simulink library "pathFollowingControllerExpStateMachineOpenWater_cl"  (R2020a)
settings: Solver=VariableStepAuto  StartTime=0.0  StopTime=10.0  RelTol=1e-3
undefined symbols (not defined in the file or in its folder): a, bScale, courseFollowExp, courseFollowExp_cl, elevatorOL, env, FLIGHTCONTROLLER, fltCtrl, initializeBussesFromBlock, maxBank, perpErrValue, rollMomentKp, rollMomentTau, tanRollKp, tanRollTau, vAppGain, vhcl, vSat, yawMomentKp
libraries: simulink x6, angleBtw2Vecs_ul x4, pathGeometry_ul x3, filteredPIDController_ul x3, eulAng2RotMat_ul x2, tanFrameProjection_ul x2, vectorNormalizer_ul x2, velocityAngle_ul x2, stopwatch_ul x1, dspsigops x1, ctrlAllocMatrixExp_cl x1, vrlib x1
settings Model: Creator=jldanie5  LastModifiedBy=andre
settings DataIOCC: ReturnWorkspaceOutputs=off
settings DebuggingCC: ArithmeticOperatorsInVariantConditions=warning
settings SFSimCC: CustomCodeUndefinedFunction=UseInterfaceOnly

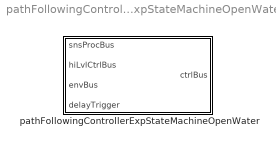
== system pathFollowingControllerExpStateMachineOpenWater_cl ==
  pathFollowingControllerExpStateMachineOpenWater : Subsystem  LoadFcn=initializeBussesFromBlock(gcb)  InitFcn=initializeBussesFromBlock(gcb)  StartFcn=initializeBussesFromBlock(gcb)  VariantControl=strcmpi(FLIGHTCONTROLLER,'pathFollowingControllerMantaBandLin')  mask{initPosForInitSStar=vhcl.initPosVecGnd.Value, fluidDensity=env.water.density.Value, pathCtrl=fltCtrl, aeroStruct=vhcl.struct('OCT.aeroSurf'), thrAttach=vhcl.rBridle_LE.Value, vhcl=vhcl}
      mask prompts: initPosForInitSStar "Initial Position"; fluidDensity "Fluid Density"; pathCtrl "Controller"; aeroStruct "Aerodynamic Structure"; thrAttach "Tether Attach Point"; vhcl "Vehicle"
      settings: MinAlgLoopOccurrences=on
      mask DialogControl Container3 Prompt: courseFollow Params
      mask DialogControl Container4 Prompt: setpointToOutput Params

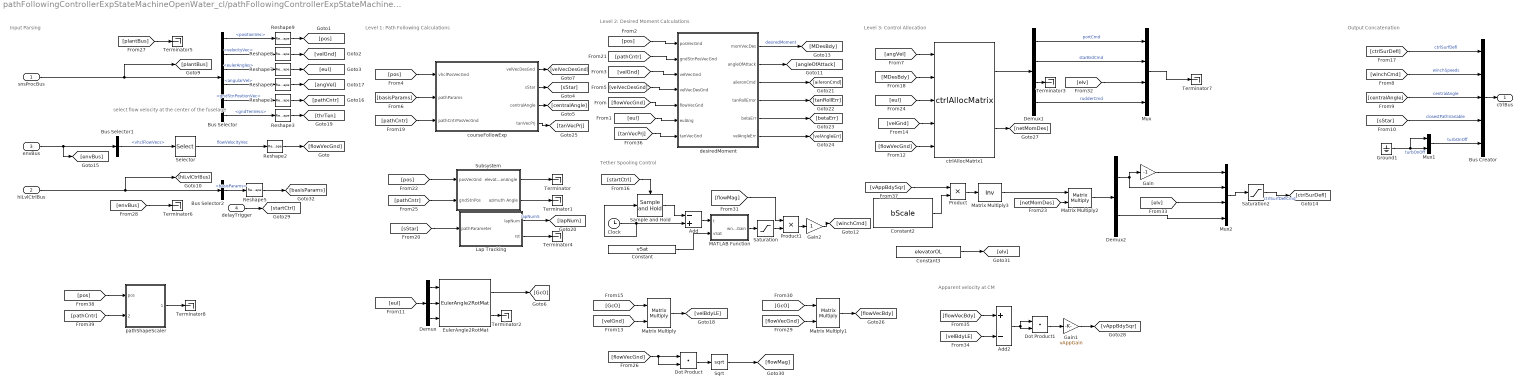
== system pathFollowingControllerExpStateMachineOpenWater_cl/pathFollowingControllerExpStateMachineOpenWater ==
  note: select flow velocity at the center of the fuselage
  note: Level 3: Control Allocation
  note: Output Concatenation
  note: Tether Spooling Control
  note: Level 2: Desired Moment Calculations
  note: Level 1: Path Following Calculations
  note: Input Parsing
  note: Apparent velocity at CM
  snsProcBus : Inport  OutDataTypeStr=Bus: sensorsProcessingBus
  hiLvlCtrlBus : Inport  Port=2  OutDataTypeStr=Bus: hiLvlCtrlBus
  envBus : Inport  Port=3  OutDataTypeStr=Bus: envBus
  delayTrigger : Inport  Port=4
  Add : Sum  Inputs=-+
  Add2 : Sum  Inputs=+-
  Bus Creator : BusCreator  Inputs=5  OutDataTypeStr=Bus: fltCtrlBus
      settings: InheritFromInputs=off
  Bus Selector : BusSelector  OutputSignals=positionVec,velocityVec,eulerAngles,angularVel,gndStnPositionVec,gndTenVecs
  Bus Selector1 : BusSelector  OutputSignals=vhclFlowVecs
  Bus Selector2 : BusSelector  OutputSignals=basisParams
  Clock : Clock
  Constant : Constant  Value=vSat
  Constant2 : Constant  Value=bScale
  Constant3 : Constant  Value=elevatorOL
  Demux : Demux  Outputs=3
  Demux1 : Demux
  Demux2 : Demux  Outputs=2
  Dot Product : DotProduct  InputSameDT=on  OutDataTypeStr=Inherit: Inherit via internal rule
  Dot Product1 : DotProduct  InputSameDT=on  OutDataTypeStr=Inherit: Inherit via internal rule
  EulerAngle2RotMat : eulAng2RotMat_ul/EulerAngle2RotMat  SystemSampleTime=-1  Latency=0  AutoFrameSizeCalculation=off
  Gain : Gain  Gain=-1
  Gain1 : Gain  Gain=vAppGain
  Gain2 : Gain
  Ground1 : Ground
  Lap Tracking : Subsystem
  MATLAB Function : MATLAB Function  TreatAsAtomicUnit=on
  Matrix Multiply : Product  Multiplication=Matrix(*)
  Matrix Multiply1 : Product  Multiplication=Matrix(*)
  Matrix Multiply2 : Product  Multiplication=Matrix(*)
  Matrix Multiply3 : Product  Inputs=/  Multiplication=Matrix(*)
  Mux : Mux
  Mux1 : Mux  Inputs=2
  Mux2 : Mux
  Product : Product
  Product1 : Product
  Reshape{1..3,5..9} (8 alike) : Reshape  OutputDimensionality=Column vector (2-D)
  Sample and Hold : dspsigops/Sample and Hold  trig=Rising edge  initCond=0  latchinput=off
  Saturation : Saturate  UpperLimit=fltCtrl.vSat.Value  LowerLimit=0
  Saturation2 : Saturate  UpperLimit=pathCtrl.controlSigMax.upperLimit.Value  LowerLimit=pathCtrl.controlSigMax.lowerLimit.Value
  Selector : Selector  NumberOfDimensions=2  InputPortWidth=3  IndexOptions=Select all,Index vector (dialog)  Indices=[1 3],5  OutputSizes=1,1
  Sqrt : Sqrt  SaturateOnIntegerOverflow=on
  Subsystem : Subsystem
  Terminator{,1..8} (9 alike) : Terminator
  courseFollowExp : Subsystem  AncestorBlock=courseFollowExp_cl/courseFollowExp
  ctrlAllocMatrix1 : ctrlAllocMatrixExp_cl/ctrlAllocMatrix  aeroStruct=vhcl.struct('OCT.aeroSurf')  fluidDensity=fluidDensity
  desiredMoment : Subsystem
  pathShapeScaler : Subsystem
  ctrlBus : Outport  OutDataTypeStr=Bus: fltCtrlBus  VectorParamsAs1DForOutWhenUnconnected=off
  wires:
  Bus Selector/6 -> Reshape3/1  "<gndTenVecs>"
  Reshape3/1 -> [thrTen]
  courseFollowExp/1(velVecDesGnd) -> [velVecDesGnd]
  snsProcBus/1 -> Bus Selector/1, [plantBus]
  Bus Selector/2 -> Reshape8/1  "<velocityVec>"
  Bus Selector/1 -> Reshape9/1  "<positionVec>"
  Bus Selector/3 -> Reshape7/1  "<eulerAngles>"
  [pos] -> courseFollowExp/1("vhclPosVecGnd ")
  Bus Creator/1 -> ctrlBus/1
  [winchCmd] -> Bus Creator/2  "winchSpeeds"
  courseFollowExp/2(sStar) -> [sStar]
  hiLvlCtrlBus/1 -> [hiLvlCtrlBus], Bus Selector2/1
  [centralAngle] -> Bus Creator/3  "centralAngle"
  [sStar] -> Bus Creator/4  "closestPathVariable"
  courseFollowExp/3(centralAngle) -> [centralAngle]
  desiredMoment/1(momVecDes) -> [MDesBdy]  "desiredMoment"
  Bus Selector/4 -> Reshape6/1  "<angularVel>"
  [angVel] -> ctrlAllocMatrix1/1
  Demux1/3 -> Terminator3/1
  Demux1/1 -> Mux/1  "portCmd"
  Demux1/2 -> Mux/2  "starBrdCmd"
  ctrlAllocMatrix1/1 -> Demux1/1
  [ctrlSurDefl] -> Bus Creator/1  "ctrlSurfDefl"
  Bus Selector2/1 -> Reshape5/1  "<basisParams>"
  Reshape5/1 -> [basisParams]
  Saturation2/1 -> [ctrlSurDefl]  "ctrlSurfDeflCmd"
  Reshape2/1 -> [flowVecGnd]
  Reshape6/1 -> [angVel]
  Reshape7/1 -> [eul]
  Reshape8/1 -> [velGnd]
  Reshape9/1 -> [pos]
  Selector/1 -> Reshape2/1  "flowVelocityVec"
  envBus/1 -> [envBus], Bus Selector1/1
  Bus Selector1/1 -> Selector/1  "<vhclFlowVecs>"
  Reshape1/1 -> [pathCntr]
  Bus Selector/5 -> Reshape1/1  "<gndStnPositionVec>"
  [pathCntr] -> courseFollowExp/3(pathCntrPosVecGnd)
  [pos] -> desiredMoment/1(posVecGnd)
  [pathCntr] -> desiredMoment/2(gndStnPosVecGnd)
  [velGnd] -> desiredMoment/3(velVecGnd)
  [velVecDesGnd] -> desiredMoment/4(velVecDesGnd)
  [eul] -> desiredMoment/6(eulAng)
  [flowVecGnd] -> desiredMoment/5(flowVecGnd)
  [basisParams] -> courseFollowExp/2(pathParams)
  Demux1/4 -> Mux/4  "rudderCmd"
  Mux1/1 -> Bus Creator/5  "turbOnOff"
  [pos] -> Subsystem/1(posVecGnd)
  Subsystem/1(elevationAngle) -> Terminator/1
  Subsystem/2(azimuth Angle) -> Terminator1/1
  [elv] -> Mux/3
  desiredMoment/2(angleOfAttack) -> [angleOfAttack]
  [sStar] -> Lap Tracking/1(pathParameter)
  Lap Tracking/2(rst) -> Terminator4/1
  Lap Tracking/1(lapNum) -> [lapNum]  "lapNumS"
  [plantBus] -> Terminator5/1
  [envBus] -> Terminator6/1
  Constant/1 -> MATLAB Function/2(vSat)
  desiredMoment/3(aileronCmd) -> [aileronCmd]
  Mux/1 -> Terminator7/1
  desiredMoment/4(tanRollError) -> [tanRollErr]
  desiredMoment/5(betaErr) -> [betaErr]
  desiredMoment/6(velAngleErr) -> [velAngleErr]
  courseFollowExp/4(tanVecPrj) -> [tanVecPrj]
  [tanVecPrj] -> desiredMoment/7(tanVecGnd)
  [eul] -> ctrlAllocMatrix1/3
  [flowVecGnd] -> ctrlAllocMatrix1/5
  [MDesBdy] -> ctrlAllocMatrix1/2
  [pathCntr] -> Subsystem/2(gndStnPos)
  Ground1/1 -> Mux1/1, Mux1/2  "turbOnOff"
  [eul] -> Demux/1
  Demux/2 -> EulerAngle2RotMat/2
  Demux/1 -> EulerAngle2RotMat/1
  Demux/3 -> EulerAngle2RotMat/3
  EulerAngle2RotMat/2 -> Terminator2/1
  EulerAngle2RotMat/1 -> [GcO]
  [velGnd] -> Matrix Multiply/2
  [GcO] -> Matrix Multiply/1
  Matrix Multiply/1 -> [velBdyLE]
  Matrix Multiply1/1 -> [flowVecBdy]
  [GcO] -> Matrix Multiply1/1
  [flowVecGnd] -> Matrix Multiply1/2
  Constant2/1 -> Product/2
  Matrix Multiply2/1 -> Demux2/1
  Demux2/1 -> Mux2/2, Gain/1
  Gain/1 -> Mux2/1
  [elv] -> Mux2/3
  Demux2/2 -> Mux2/4
  Add2/1 -> Dot Product1/1, Dot Product1/2
  [flowVecBdy] -> Add2/1
  [velBdyLE] -> Add2/2
  Product/1 -> Matrix Multiply3/1
  Matrix Multiply3/1 -> Matrix Multiply2/1
  ctrlAllocMatrix1/2 -> [netMomDes]
  Dot Product1/1 -> Gain1/1
  [netMomDes] -> Matrix Multiply2/2
  [vAppBdySqr] -> Product/1
  Gain1/1 -> [vAppBdySqr]
  delayTrigger/1 -> [startCtrl]
  [startCtrl] -> Sample and Hold/Trigger
  Clock/1 -> Add/2, Sample and Hold/1
  Sample and Hold/1 -> Add/1
  Add/1 -> MATLAB Function/1(t)
  [flowVecGnd] -> Dot Product/2, Dot Product/1
  Dot Product/1 -> Sqrt/1
  Sqrt/1 -> [flowMag]
  MATLAB Function/1(wnchGain) -> Saturation/1
  [flowMag] -> Product1/1
  Product1/1 -> Gain2/1
  Constant3/1 -> [elv]
  Gain2/1 -> [winchCmd]
  Saturation/1 -> Product1/2
  [pos] -> pathShapeScaler/1(pos)
  [pathCntr] -> pathShapeScaler/2(pathCntr)
  pathShapeScaler/1(basisParams) -> Terminator8/1
  Mux2/1 -> Saturation2/1
  [velGnd] -> ctrlAllocMatrix1/4

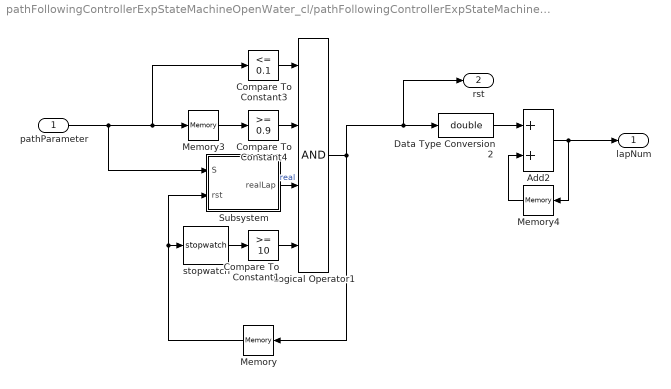
== system pathFollowingControllerExpStateMachineOpenWater_cl/pathFollowingControllerExpStateMachineOpenWater/Lap Tracking ==
  pathParameter : Inport
  Add2 : Sum
  Compare To Constant1 : simulink/Logic and Bit Operations/Compare To Constant  relop=>=  const=10  OutDataTypeStr=boolean
  Compare To Constant3 : simulink/Logic and Bit Operations/Compare To Constant  relop=<=  const=0.1  OutDataTypeStr=boolean
  Compare To Constant4 : simulink/Logic and Bit Operations/Compare To Constant  relop=>=  const=0.9  OutDataTypeStr=boolean
  Data Type Conversion2 : DataTypeConversion  OutDataTypeStr=double
  Logical Operator1 : Logic  Inputs=4  AllPortsSameDT=off  OutDataTypeStr=boolean
  Memory : Memory  InitialCondition=false
  Memory3 : Memory
  Memory4 : Memory
  Subsystem : Subsystem
  stopwatch : stopwatch_ul/stopwatch  SystemSampleTime=-1  Latency=0  AutoFrameSizeCalculation=off
  lapNum : Outport  VectorParamsAs1DForOutWhenUnconnected=off
  rst : Outport  Port=2  VectorParamsAs1DForOutWhenUnconnected=off
  wires:
  Compare To Constant3/1 -> Logical Operator1/1
  Memory3/1 -> Compare To Constant4/1
  Data Type Conversion2/1 -> Add2/1
  Logical Operator1/1 -> rst/1, Data Type Conversion2/1, Memory/1
  Memory4/1 -> Add2/2
  Add2/1 -> lapNum/1, Memory4/1
  Compare To Constant4/1 -> Logical Operator1/2
  pathParameter/1 -> Subsystem/1(S), Compare To Constant3/1, Memory3/1
  stopwatch/1 -> Compare To Constant1/1
  Memory/1 -> Subsystem/2(rst), stopwatch/1
  Compare To Constant1/1 -> Logical Operator1/4
  Subsystem/1(realLap) -> Logical Operator1/3  "real"

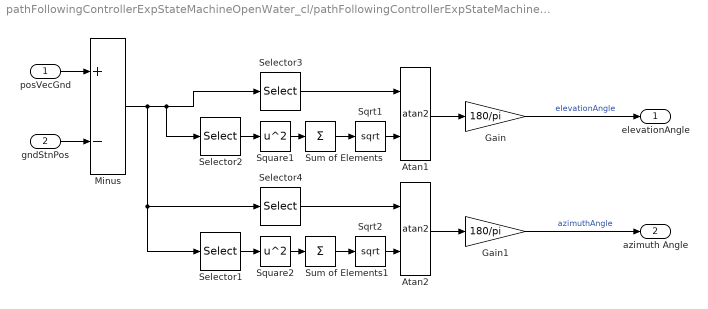
== system pathFollowingControllerExpStateMachineOpenWater_cl/pathFollowingControllerExpStateMachineOpenWater/Subsystem ==
  posVecGnd : Inport
  gndStnPos : Inport  Port=2
  Atan1 : Trigonometry  Operator=atan2
  Atan2 : Trigonometry  Operator=atan2
  Gain : Gain  Gain=180/pi
  Gain1 : Gain  Gain=180/pi
  Minus : Sum  Inputs=+-
  Selector1 : Selector  InputPortWidth=3  IndexOptions=Index vector (dialog)  Indices=1  OutputSizes=1
  Selector2 : Selector  InputPortWidth=3  IndexOptions=Index vector (dialog)  Indices=[1 2]  OutputSizes=1
  Selector3 : Selector  InputPortWidth=3  IndexOptions=Index vector (dialog)  Indices=3  OutputSizes=1
  Selector4 : Selector  InputPortWidth=3  IndexOptions=Index vector (dialog)  Indices=2  OutputSizes=1
  Sqrt1 : Sqrt  SaturateOnIntegerOverflow=on
  Sqrt2 : Sqrt  SaturateOnIntegerOverflow=on
  Square1 : Math  Operator=square  SignedPower=on  SaturateOnIntegerOverflow=on
  Square2 : Math  Operator=square  SignedPower=on  SaturateOnIntegerOverflow=on
  Sum of Elements : Sum  Inputs=+
  Sum of Elements1 : Sum  Inputs=+
  elevationAngle : Outport
  azimuth Angle : Outport  Port=2
  wires:
  Gain1/1 -> azimuth Angle/1  "azimuthAngle"
  Selector4/1 -> Atan2/1
  Sqrt2/1 -> Atan2/2
  Selector1/1 -> Square2/1
  Sum of Elements1/1 -> Sqrt2/1
  Square2/1 -> Sum of Elements1/1
  Atan2/1 -> Gain1/1
  Gain/1 -> elevationAngle/1  "elevationAngle"
  Selector2/1 -> Square1/1
  Atan1/1 -> Gain/1
  Sum of Elements/1 -> Sqrt1/1
  Selector3/1 -> Atan1/1
  Square1/1 -> Sum of Elements/1
  Sqrt1/1 -> Atan1/2
  posVecGnd/1 -> Minus/1
  gndStnPos/1 -> Minus/2
  Minus/1 -> Selector4/1, Selector1/1, Selector2/1, Selector3/1

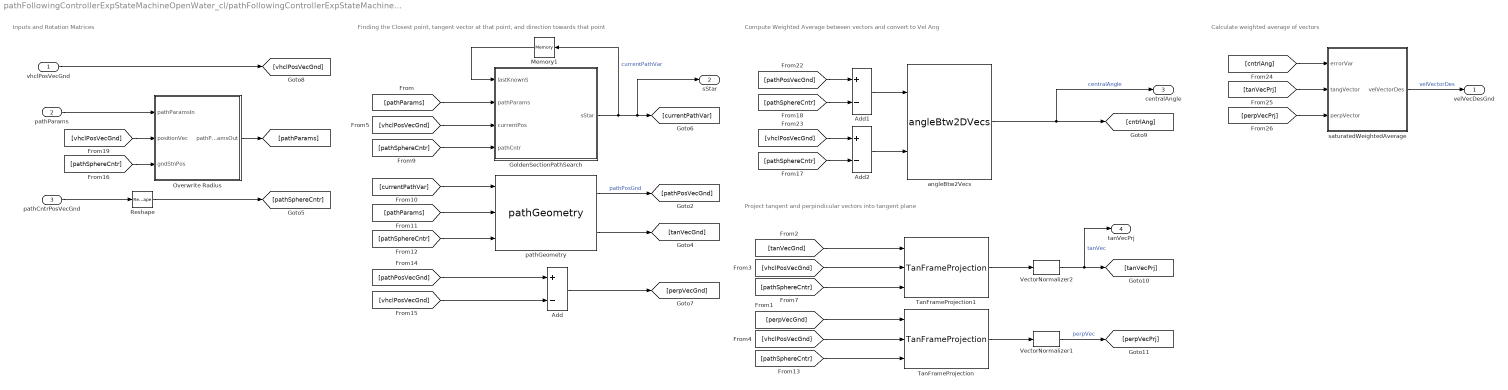
== system pathFollowingControllerExpStateMachineOpenWater_cl/pathFollowingControllerExpStateMachineOpenWater/courseFollowExp ==
  note: Finding the Closest point, tangent vector at that point, and direction towards that point
  note: Inputs and Rotation Matrices
  note: Compute Weighted Average between vectors and convert to Vel Ang
  note: Project tangent and perpindicular vectors into tangent plane
  note: Calculate weighted average of vectors
  "vhclPosVecGnd " : Inport
  pathParams : Inport  Port=2
  pathCntrPosVecGnd : Inport  Port=3
  Add : Sum  Inputs=+-
  Add1 : Sum  Inputs=+-
  Add2 : Sum  Inputs=+-
  GoldenSectionPathSearch : Subsystem  TreatAsAtomicUnit=on
  Memory1 : Memory  InitialCondition=pathCtrl.initPathVar.Value
  Overwrite Radius : Subsystem
  Reshape : Reshape  OutputDimensionality=Column vector (2-D)
  TanFrameProjection : tanFrameProjection_ul/TanFrameProjection  SystemSampleTime=-1  Latency=0  AutoFrameSizeCalculation=off
  TanFrameProjection1 : tanFrameProjection_ul/TanFrameProjection  SystemSampleTime=-1  Latency=0  AutoFrameSizeCalculation=off
  VectorNormalizer1 : vectorNormalizer_ul/VectorNormalizer   SystemSampleTime=-1  Latency=0  AutoFrameSizeCalculation=off
  VectorNormalizer2 : vectorNormalizer_ul/VectorNormalizer   SystemSampleTime=-1  Latency=0  AutoFrameSizeCalculation=off
  angleBtw2Vecs : angleBtw2Vecs_ul/angleBtw2DVecs  SystemSampleTime=-1  Latency=0  AutoFrameSizeCalculation=off
  pathGeometry : pathGeometry_ul/pathGeometry  SystemSampleTime=-1  Latency=0  AutoFrameSizeCalculation=off
  saturatedWeightedAverage : Subsystem  mask{error_upper_lim=perpErrValue}
      mask prompts: error_upper_lim "Value of Error yielding 100% perpendicular"
  velVecDesGnd : Outport  VectorParamsAs1DForOutWhenUnconnected=off
  sStar : Outport  Port=2  VectorParamsAs1DForOutWhenUnconnected=off
  centralAngle : Outport  Port=3  VectorParamsAs1DForOutWhenUnconnected=off
  tanVecPrj : Outport  Port=4
  wires:
  saturatedWeightedAverage/1("velVectorDes ") -> velVecDesGnd/1  "velVectorDes"
  [perpVecPrj] -> saturatedWeightedAverage/3("perpVector ")
  [tanVecPrj] -> saturatedWeightedAverage/2(tangVector)
  [cntrlAng] -> saturatedWeightedAverage/1("errorVar ")
  [pathSphereCntr] -> TanFrameProjection/3
  [pathSphereCntr] -> TanFrameProjection1/3
  [vhclPosVecGnd] -> TanFrameProjection/2
  [vhclPosVecGnd] -> TanFrameProjection1/2
  [tanVecGnd] -> TanFrameProjection1/1
  [perpVecGnd] -> TanFrameProjection/1
  [vhclPosVecGnd] -> Overwrite Radius/2(positionVec)
  [pathSphereCntr] -> Overwrite Radius/3(gndStnPos)
  Add2/1 -> angleBtw2Vecs/2
  Add1/1 -> angleBtw2Vecs/1
  [pathSphereCntr] -> Add1/2
  [pathSphereCntr] -> Add2/2
  [pathSphereCntr] -> GoldenSectionPathSearch/4(pathCntr)
  [pathSphereCntr] -> pathGeometry/3
  Reshape/1 -> [pathSphereCntr]
  pathCntrPosVecGnd/1 -> Reshape/1
  Overwrite Radius/1(pathParamsOut) -> [pathParams]
  pathParams/1 -> Overwrite Radius/1(pathParamsIn)
  TanFrameProjection/1 -> VectorNormalizer1/1
  pathGeometry/2 -> [tanVecGnd]
  [pathPosVecGnd] -> Add/1
  [vhclPosVecGnd] -> Add/2
  Add/1 -> [perpVecGnd]
  Memory1/1 -> GoldenSectionPathSearch/1(lastKnownS)
  GoldenSectionPathSearch/1(sStar) -> [currentPathVar], sStar/1, Memory1/1  "currentPathVar"
  [pathParams] -> GoldenSectionPathSearch/2(pathParams)
  TanFrameProjection1/1 -> VectorNormalizer2/1
  [currentPathVar] -> pathGeometry/1
  [vhclPosVecGnd] -> Add2/1
  angleBtw2Vecs/1 -> centralAngle/1, [cntrlAng]  "centralAngle"
  VectorNormalizer1/1 -> [perpVecPrj]  "perpVec"
  [pathParams] -> pathGeometry/2
  pathGeometry/1 -> [pathPosVecGnd]  "pathPosGnd"
  "vhclPosVecGnd "/1 -> [vhclPosVecGnd]
  [vhclPosVecGnd] -> GoldenSectionPathSearch/3(currentPos)
  VectorNormalizer2/1 -> [tanVecPrj], tanVecPrj/1  "tanVec"
  [pathPosVecGnd] -> Add1/1

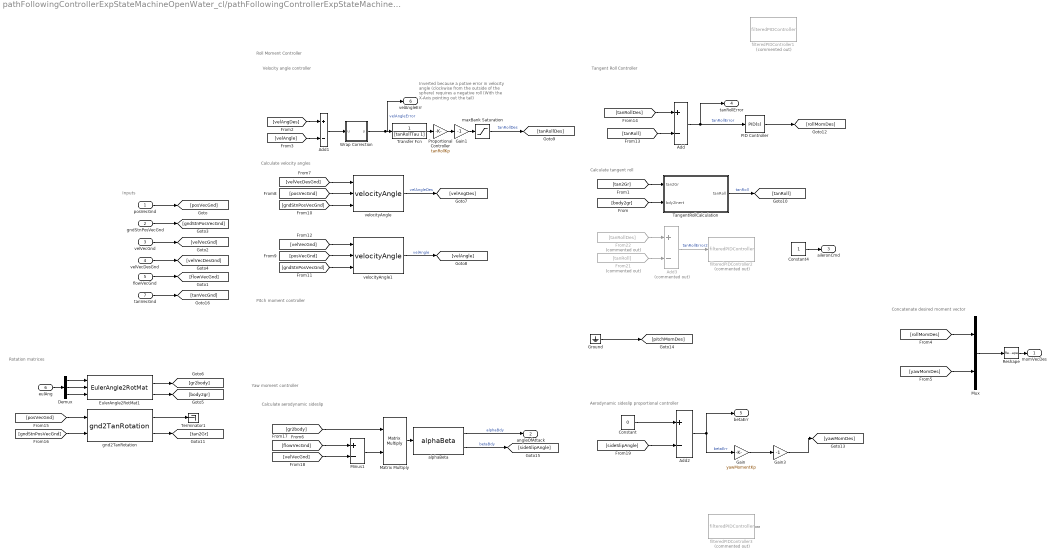
== system pathFollowingControllerExpStateMachineOpenWater_cl/pathFollowingControllerExpStateMachineOpenWater/desiredMoment ==
  note: Yaw moment controller
  note: Pitch moment controller
  note: Inverted because a potive error
      | in velocity angle (clockwise from the
      | outside of the sphere) requires a negative
      | roll (With the X-Axis pointing out the tail)
  note: Velocity angle controller
  note: Inputs
  note: Rotation matrices
  note: Calculate velocity angles
  note: Calculate tangent roll
  note: Tangent Roll Controller
  note: Concatenate desired moment vector
  note: Roll Moment Controller
  note: Aerodynamic sideslip proportional controller
  note: Calculate aerodynamic sideslip
  posVecGnd : Inport
  gndStnPosVecGnd : Inport  Port=2
  velVecGnd : Inport  Port=3
  velVecDesGnd : Inport  Port=4
  flowVecGnd : Inport  Port=5
  eulAng : Inport  Port=6
  tanVecGnd : Inport  Port=7
  Add : Sum  Inputs=+-
  Add1 : Sum  Inputs=+-
  Add2 : Sum  Inputs=+-
  Add3 : Sum  Commented=on  Inputs=+-
  Constant : Constant  Value=0
  Constant4 : Constant
  Demux : Demux  Outputs=3
  EulerAngle2RotMat1 : eulAng2RotMat_ul/EulerAngle2RotMat  SystemSampleTime=-1  Latency=0  AutoFrameSizeCalculation=off
  From21 : From  Commented=on  GotoTag=tanRoll
  From22 : From  Commented=on  GotoTag=tanRollDes
  Gain : Gain  Gain=yawMomentKp
  Gain1 : Gain  Gain=-1
  Gain3 : Gain  Gain=-1
  Ground : Ground
  Matrix Multiply : Product  Multiplication=Matrix(*)
  Minus1 : Sum  Inputs=+-
  Mux : Mux  Inputs=2
  PID Controller : simulink/Continuous/PID Controller  Controller=PID  Form=Parallel  TimeDomain=Continuous-time  UseExternalTs=off  SampleTime=-1  IntegratorMethod=Forward Euler  FilterMethod=Forward Euler  ControllerParametersSource=internal  P=rollMomentKp  I=0  D=fltCtrl.rollMoment.kd.Value  UseFilter=on  N=1/rollMomentTau  TunerSelectOption=Transfer Function Based (PID Tuner App)  InitialConditionSource=internal  InitialConditionForIntegrator=0  InitialConditionForFilter=0  DifferentiatorICPrevScaledInput=0  ExternalReset=none  TrackingMode=off  Kt=1  LimitOutput=off  UpperSaturationLimit=inf  LowerSaturationLimit=-inf  LinearizeAsGain=on  AntiWindupMode=none  Kb=1  POutMin=[]  POutMax=[]  IOutMin=[]  IOutMax=[]  DOutMin=[]  DOutMax=[]  NOutMin=[]  NOutMax=[]  SumOutMin=[]  SumOutMax=[]  SaturationOutMin=[]  SaturationOutMax=[]  PParamMin=[]  PParamMax=[]  IParamMin=[]  IParamMax=[]  DParamMin=[]  DParamMax=[]  NParamMin=[]  NParamMax=[]  KbParamMin=[]  KbParamMax=[]  KtParamMin=[]  KtParamMax=[]  KbOutMin=[]  KbOutMax=[]  KtOutMin=[]  KtOutMax=[]  IntegratorOutMin=[]  IntegratorOutMax=[]  FilterOutMin=[]  FilterOutMax=[]  SumI1OutMin=[]  SumI1OutMax=[]  SumI2OutMin=[]  SumI2OutMax=[]  SumI3OutMin=[]  SumI3OutMax=[]  SumI4OutMin=[]  SumI4OutMax=[]  SumDOutMin=[]  SumDOutMax=[]  DifferentiatorOutMin=[]  DifferentiatorOutMax=[]  FilterDiffOutCoefMin=[]  FilterDiffOutCoefMax=[]  ReciprocalOutMin=[]  ReciprocalOutMax=[]  SumDenOutMin=[]  SumDenOutMax=[]  SumNumOutMin=[]  SumNumOutMax=[]  DivideOutMin=[]  DivideOutMax=[]  UdiffTsProdOutMin=[]  UdiffTsProdOutMax=[]  NTsProdOutMin=[]  NTsProdOutMax=[]  UintegralTsProdOutMin=[]  UintegralTsProdOutMax=[]  UngainTsProdOutMin=[]  UngainTsProdOutMax=[]  IntegratorContinuousStateAttributes=''  IntegratorStateMustResolveToSignalObject=off  IntegratorRTWStateStorageClass=Auto  FilterContinuousStateAttributes=''  FilterStateMustResolveToSignalObject=off  FilterRTWStateStorageClass=Auto  ParallelPVariant=InternalParameters  IdealPVariant=Disabled  IVariant=InternalParameters  DVariant=InternalParameters  IntegratorVariant=Continuous  SatVariant=Disabled  AWVariant=Passthrough  PCopyVariant=Disabled  TRVariant=Disabled  FdbkBlocksVariant=Forward  IdealPFdbkVariant=Disabled  SatFdbkVariant=Disabled  DerivativeFilterVariant=ContFilter  NVariant=InternalParameters  NCopyVariant=Disabled  FilterICVariant=InternalICsFilter  IntegratorICVariant=InternalICs  ExternalResetVariant=Disabled  TRSumVariant=Passthrough  SumFdbkVariant=Disabled  SumVariant=Sum_PID  TsampFilterVariant=InternalTs  TsampNgainVariant=Passthrough  TsampIntegralVariant=Passthrough
  Proportional Controller : Gain  Gain=tanRollKp
  Reshape : Reshape  OutputDimensionality=Column vector (2-D)
  TangentRollCalculation : Subsystem
  Terminator1 : Terminator
  Transfer Fcn : TransferFcn  Denominator=[tanRollTau 1]
  Wrap Correction : Subsystem
  alphaBeta : alphaBeta_ul/alphaBeta  SystemSampleTime=-1  Latency=0  AutoFrameSizeCalculation=off
  filteredPIDController1 : filteredPIDController_ul/filteredPIDController  Commented=on  kp=pathCtrl.rollMoment.kp.Value  ki=0  kd=pathCtrl.rollMoment.kd.Value  Value=pathCtrl.rollMoment.tau.Value  externalReset=none
  filteredPIDController2 : filteredPIDController_ul/filteredPIDController  Commented=on  kp=fltCtrl.rollCtrl.kp.Value  ki=fltCtrl.rollCtrl.ki.Value  kd=fltCtrl.rollCtrl.kd.Value  Value=fltCtrl.rollCtrl.tau.Value  externalReset=none
  filteredPIDController3 : filteredPIDController_ul/filteredPIDController  Commented=on  kp=pathCtrl.yawMoment.kp.Value  ki=0  kd=pathCtrl.yawMoment.kd.Value  Value=pathCtrl.yawMoment.tau.Value  externalReset=none
  gnd2TanRotation : gnd2TanRotation_ul/gnd2TanRotation  SystemSampleTime=-1  Latency=0  AutoFrameSizeCalculation=off
  maxBank Saturation : Saturate  UpperLimit=maxBank  LowerLimit=-maxBank
  velocityAngle : velocityAngle_ul/velocityAngle  SystemSampleTime=-1  Latency=0  AutoFrameSizeCalculation=off
  velocityAngle1 : velocityAngle_ul/velocityAngle  SystemSampleTime=-1  Latency=0  AutoFrameSizeCalculation=off
  momVecDes : Outport  VectorParamsAs1DForOutWhenUnconnected=off
  angleOfAttack : Outport  Port=2  VectorParamsAs1DForOutWhenUnconnected=off
  aileronCmd : Outport  Port=3  VectorParamsAs1DForOutWhenUnconnected=off
  tanRollError : Outport  Port=4
  betaErr : Outport  Port=5
  velAngleErr : Outport  Port=6
  wires:
  [yawMomDes] -> Mux/2
  gnd2TanRotation/1 -> Terminator1/1
  gnd2TanRotation/2 -> [tan2Gr]
  [gndStnPosVecGnd] -> gnd2TanRotation/2
  [posVecGnd] -> gnd2TanRotation/1
  [tanRollDes] -> Add/1
  [tanRoll] -> Add/2
  [velVecGnd] -> velocityAngle1/1
  [gndStnPosVecGnd] -> velocityAngle1/3
  [gndStnPosVecGnd] -> velocityAngle/3
  [posVecGnd] -> velocityAngle1/2
  [posVecGnd] -> velocityAngle/2
  [velVecDesGnd] -> velocityAngle/1
  [velAngle] -> Add1/2
  [velAngDes] -> Add1/1
  velocityAngle1/1 -> [velAngle]  "velAngle"
  velocityAngle/1 -> [velAngDes]  "velAngleDes"
  velVecDesGnd/1 -> [velVecDesGnd]
  gndStnPosVecGnd/1 -> [gndStnPosVecGnd]
  alphaBeta/1 -> angleOfAttack/1  "alphaBdy"
  Add2/1 -> Gain/1, betaErr/1  "betaErr"
  alphaBeta/2 -> [sideSlipAngle]  "betaBdy"
  Matrix Multiply/1 -> alphaBeta/1
  [gr2body] -> Matrix Multiply/1
  [body2gr] -> TangentRollCalculation/2(bdy2Inert)
  EulerAngle2RotMat1/1 -> [gr2body]
  EulerAngle2RotMat1/2 -> [body2gr]
  Demux/2 -> EulerAngle2RotMat1/2
  Demux/1 -> EulerAngle2RotMat1/1
  Demux/3 -> EulerAngle2RotMat1/3
  eulAng/1 -> Demux/1
  [flowVecGnd] -> Minus1/1
  [velVecGnd] -> Minus1/2
  Minus1/1 -> Matrix Multiply/2
  filteredPIDController3/1 -> ?
  TangentRollCalculation/1(tanRoll) -> [tanRoll]  "tanRoll"
  [tan2Gr] -> TangentRollCalculation/1(tan2Gr)
  flowVecGnd/1 -> [flowVecGnd]
  Add1/1 -> Wrap Correction/1(u)
  maxBank Saturation/1 -> [tanRollDes]  "tanRollDes"
  Gain1/1 -> maxBank Saturation/1
  Proportional Controller/1 -> Gain1/1
  Add/1 -> PID Controller/1, tanRollError/1  "tanRollError"
  velVecGnd/1 -> [velVecGnd]
  posVecGnd/1 -> [posVecGnd]
  Ground/1 -> [pitchMomDes]
  Transfer Fcn/1 -> Proportional Controller/1
  Add3/1 -> filteredPIDController2/1  "tanRollError2"
  From21/1 -> Add3/2
  From22/1 -> Add3/1
  tanVecGnd/1 -> [tanVecGnd]
  Wrap Correction/1(y) -> velAngleErr/1, Transfer Fcn/1  "velAngleError"
  Mux/1 -> Reshape/1
  [rollMomDes] -> Mux/1
  Gain3/1 -> [yawMomDes]
  Constant4/1 -> aileronCmd/1
  Reshape/1 -> momVecDes/1
  [sideSlipAngle] -> Add2/2
  PID Controller/1 -> [rollMomDes]
  Gain/1 -> Gain3/1
  Constant/1 -> Add2/1

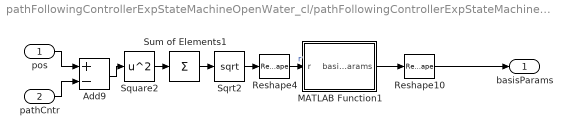
== system pathFollowingControllerExpStateMachineOpenWater_cl/pathFollowingControllerExpStateMachineOpenWater/pathShapeScaler ==
  pos : Inport
  pathCntr : Inport  Port=2
  Add9 : Sum  Inputs=+-
  MATLAB Function1 : MATLAB Function  TreatAsAtomicUnit=on
  Reshape10 : Reshape  OutputDimensionality=Column vector (2-D)
  Reshape4 : Reshape
  Sqrt2 : Sqrt  SaturateOnIntegerOverflow=on
  Square2 : Math  Operator=square  SaturateOnIntegerOverflow=on
  Sum of Elements1 : Sum  Inputs=+
  basisParams : Outport
  wires:
  Sum of Elements1/1 -> Sqrt2/1
  Square2/1 -> Sum of Elements1/1
  MATLAB Function1/1(basisParams) -> Reshape10/1
  pos/1 -> Add9/1
  pathCntr/1 -> Add9/2
  Sqrt2/1 -> Reshape4/1
  Reshape4/1 -> MATLAB Function1/1(r)  "r"
  Reshape10/1 -> basisParams/1
  Add9/1 -> Square2/1

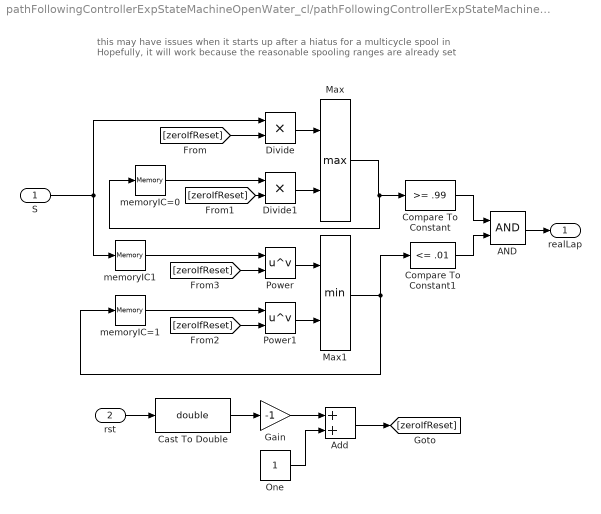
== system pathFollowingControllerExpStateMachineOpenWater_cl/pathFollowingControllerExpStateMachineOpenWater/Lap Tracking/Subsystem ==
  note: this may have issues when it starts up after a hiatus for a multicycle spool in
      | Hopefully, it will work because the reasonable spooling ranges are already set
  S : Inport
  rst : Inport  Port=2
  AND : Logic  AllPortsSameDT=off  OutDataTypeStr=boolean
  Add : Sum
  Cast To Double : DataTypeConversion  OutDataTypeStr=double
  Compare To Constant : simulink/Logic and Bit Operations/Compare To Constant  relop=>=  const=.99  OutDataTypeStr=boolean
  Compare To Constant1 : simulink/Logic and Bit Operations/Compare To Constant  relop=<=  const=.01  OutDataTypeStr=boolean
  Divide : Product  Inputs=**
  Divide1 : Product  Inputs=**
  Gain : Gain  Gain=-1
  Max : MinMax  Function=max  Inputs=2
  Max1 : MinMax  Inputs=2
  One : Constant  OutDataTypeStr=Inherit: Inherit via back propagation
  Power : Math  Operator=pow  SaturateOnIntegerOverflow=on
  Power1 : Math  Operator=pow  SaturateOnIntegerOverflow=on
  memoryIC1 : Memory  InitialCondition=1
  memoryIC=0 : Memory
  memoryIC=1 : Memory  InitialCondition=1
  realLap : Outport
  wires:
  Max1/1 -> Compare To Constant1/1, memoryIC=1/1
  rst/1 -> Cast To Double/1
  S/1 -> Divide/1, memoryIC1/1
  Gain/1 -> Add/1
  Add/1 -> [zeroIfReset]
  One/1 -> Add/2
  Divide/1 -> Max/1
  Max/1 -> memoryIC=0/1, Compare To Constant/1
  Power/1 -> Max1/1
  Power1/1 -> Max1/2
  Cast To Double/1 -> Gain/1
  Compare To Constant/1 -> AND/1
  Compare To Constant1/1 -> AND/2
  AND/1 -> realLap/1
  [zeroIfReset] -> Divide/2
  [zeroIfReset] -> Power/2
  [zeroIfReset] -> Divide1/2
  Divide1/1 -> Max/2
  memoryIC=0/1 -> Divide1/1
  [zeroIfReset] -> Power1/2
  memoryIC=1/1 -> Power1/1
  memoryIC1/1 -> Power/1

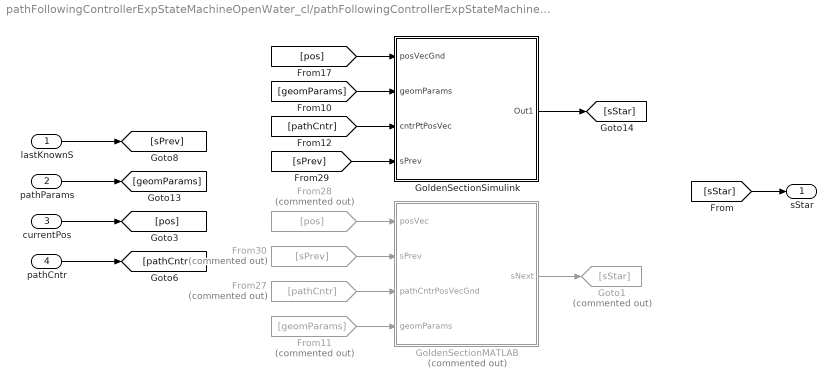
== system pathFollowingControllerExpStateMachineOpenWater_cl/pathFollowingControllerExpStateMachineOpenWater/courseFollowExp/GoldenSectionPathSearch ==
  lastKnownS : Inport
  pathParams : Inport  Port=2
  currentPos : Inport  Port=3
  pathCntr : Inport  Port=4
  From11 : From  Commented=on  GotoTag=geomParams
  From27 : From  Commented=on  GotoTag=pathCntr
  From28 : From  Commented=on  GotoTag=pos
  From30 : From  Commented=on  GotoTag=sPrev
  GoldenSectionMATLAB : MATLAB Function  Commented=on  TreatAsAtomicUnit=on  mask{geomFunc=pathCtrl, searchWidth=0.1, pathVarTol=1e-5}
  GoldenSectionSimulink : Subsystem
  Goto1 : Goto  Commented=on  GotoTag=sStar
  sStar : Outport  InitialOutput=pathCtrl.initPathVar.Value  VectorParamsAs1DForOutWhenUnconnected=off
  wires:
  GoldenSectionSimulink/1(Out1) -> [sStar]
  [sPrev] -> GoldenSectionSimulink/4(sPrev)
  [pathCntr] -> GoldenSectionSimulink/3(cntrPtPosVec)
  [geomParams] -> GoldenSectionSimulink/2(geomParams)
  [pos] -> GoldenSectionSimulink/1(posVecGnd)
  [sStar] -> sStar/1
  lastKnownS/1 -> [sPrev]
  From27/1 -> GoldenSectionMATLAB/3(pathCntrPosVecGnd)
  From30/1 -> GoldenSectionMATLAB/2(sPrev)
  From28/1 -> GoldenSectionMATLAB/1(posVec)
  From11/1 -> GoldenSectionMATLAB/4(geomParams)
  GoldenSectionMATLAB/1(sNext) -> Goto1/1
  pathCntr/1 -> [pathCntr]
  pathParams/1 -> [geomParams]
  currentPos/1 -> [pos]

== system pathFollowingControllerExpStateMachineOpenWater_cl/pathFollowingControllerExpStateMachineOpenWater/courseFollowExp/Overwrite Radius ==
  note: subsystem overwrites the 5th basis parameter with the current radius
      | so that the downstream blocks calculate the path geomatry at the current radius.
  pathParamsIn : Inport
  positionVec : Inport  Port=2
  gndStnPos : Inport  Port=3
  Add : Sum  Inputs=+-
  Assignment : Assignment  NumberOfDimensions=2  DiagnosticForDimensions=Warning  IndexOptions=Index vector (dialog),Assign all  Indices=5,5  OutputSizes=1,1
  Dot Product : DotProduct  InputSameDT=on  OutDataTypeStr=Inherit: Inherit via internal rule
  Sqrt : Sqrt  SaturateOnIntegerOverflow=on
  pathParamsOut : Outport  VectorParamsAs1DForOutWhenUnconnected=off
  wires:
  gndStnPos/1 -> Add/2
  positionVec/1 -> Add/1
  pathParamsIn/1 -> Assignment/1
  Sqrt/1 -> Assignment/2
  Assignment/1 -> pathParamsOut/1
  Dot Product/1 -> Sqrt/1
  Add/1 -> Dot Product/1, Dot Product/2

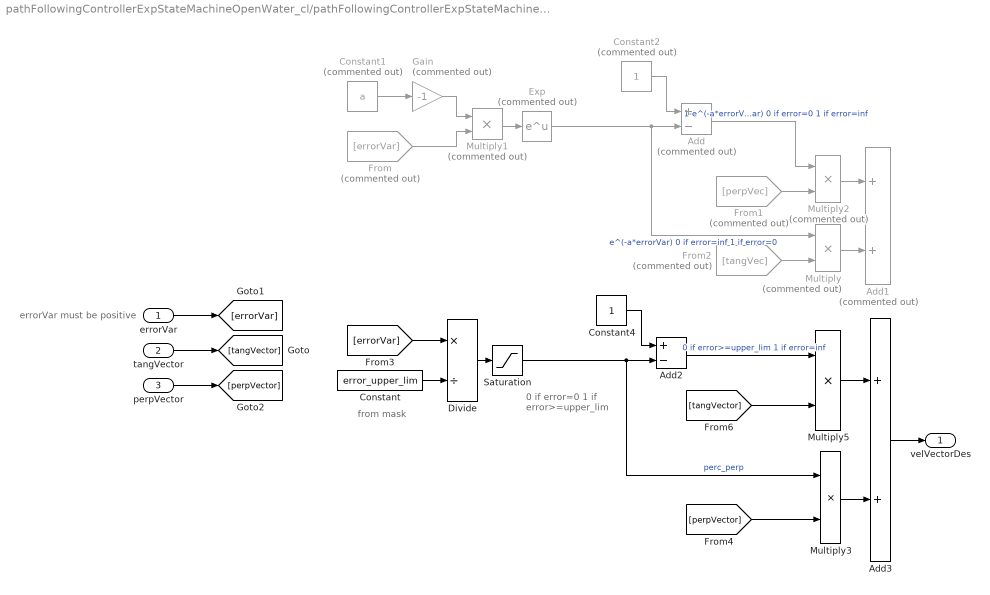
== system pathFollowingControllerExpStateMachineOpenWater_cl/pathFollowingControllerExpStateMachineOpenWater/courseFollowExp/saturatedWeightedAverage ==
  note: 0 if error=0
      | 1 if error>=upper_lim
  note: from mask
  note: errorVar must be positive
  "errorVar " : Inport
  tangVector : Inport  Port=2
  "perpVector " : Inport  Port=3
  Add : Sum  Commented=on  Inputs=+-
  Add1 : Sum  Commented=on
  Add2 : Sum  Inputs=+-
  Add3 : Sum
  Constant : Constant  Value=error_upper_lim
  Constant1 : Constant  Commented=on  Value=a
  Constant2 : Constant  Commented=on
  Constant4 : Constant
  Divide : Product  Inputs=*/
  Exp : Math  Commented=on  SignedPower=on  SaturateOnIntegerOverflow=on
  From : From  Commented=on  GotoTag=errorVar
  From1 : From  Commented=on  GotoTag=perpVec
  From2 : From  Commented=on  GotoTag=tangVec
  Gain : Gain  Commented=on  Gain=-1
  Multiply : Product  Commented=on
  Multiply1 : Product  Commented=on
  Multiply2 : Product  Commented=on
  Multiply3 : Product
  Multiply5 : Product
  Saturation : Saturate  UpperLimit=1  LowerLimit=0
  "velVectorDes " : Outport  VectorParamsAs1DForOutWhenUnconnected=off
  wires:
  tangVector/1 -> [tangVector]
  Constant1/1 -> Gain/1
  Gain/1 -> Multiply1/1
  Multiply1/1 -> Exp/1
  Exp/1 -> Multiply/1, Add/2  "e^(-a*errorVar) 0 if error=inf 1 if error=0"
  Constant2/1 -> Add/1
  Add/1 -> Multiply2/1  "1-e^(-a*errorVar) 0 if error=0 1 if error=inf"
  "errorVar "/1 -> [errorVar]
  "perpVector "/1 -> [perpVector]
  From/1 -> Multiply1/2
  Multiply2/1 -> Add1/1
  Multiply/1 -> Add1/2
  From1/1 -> Multiply2/2
  From2/1 -> Multiply/2
  Constant4/1 -> Add2/1
  Saturation/1 -> Multiply3/1, Add2/2  "perc_perp"
  Add3/1 -> "velVectorDes "/1
  Multiply3/1 -> Add3/2
  Multiply5/1 -> Add3/1
  Add2/1 -> Multiply5/1  "0 if error>=upper_lim 1 if error=inf"
  [errorVar] -> Divide/1
  Constant/1 -> Divide/2
  Divide/1 -> Saturation/1
  [tangVector] -> Multiply5/2
  [perpVector] -> Multiply3/2

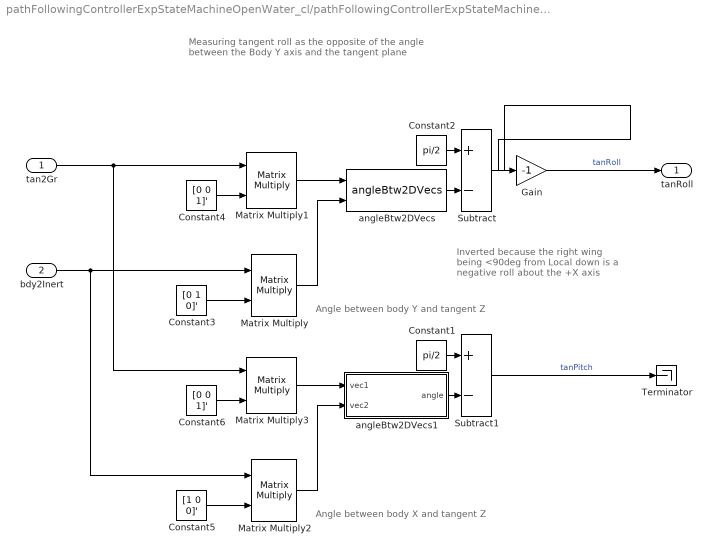
== system pathFollowingControllerExpStateMachineOpenWater_cl/pathFollowingControllerExpStateMachineOpenWater/desiredMoment/TangentRollCalculation ==
  note: Angle between body X and tangent Z
  note: Inverted because the right wing
      | being <90deg from Local down
      | is a negative roll about the +X axis
  note: Angle between body Y and tangent Z
  note: Measuring tangent roll as the opposite
      | of the angle between the Body Y axis
      | and the tangent plane
  tan2Gr : Inport
  bdy2Inert : Inport  Port=2
  Constant1 : Constant  Value=pi/2
  Constant2 : Constant  Value=pi/2
  Constant3 : Constant  Value=[0 1 0]'
  Constant4 : Constant  Value=[0 0 1]'
  Constant5 : Constant  Value=[1 0 0]'
  Constant6 : Constant  Value=[0 0 1]'
  Gain : Gain  Gain=-1
  Matrix Multiply{,1..3} (4 alike) : Product  Multiplication=Matrix(*)
  Subtract : Sum  Inputs=+-
  Subtract1 : Sum  Inputs=+-
  Terminator : Terminator
  angleBtw2DVecs : angleBtw2Vecs_ul/angleBtw2DVecs  SystemSampleTime=-1  Latency=0  AutoFrameSizeCalculation=off
  angleBtw2DVecs1 : Subsystem
  tanRoll : Outport  VectorParamsAs1DForOutWhenUnconnected=off
  wires:
  Constant5/1 -> Matrix Multiply2/2
  angleBtw2DVecs1/1(angle) -> Subtract1/2
  Constant1/1 -> Subtract1/1
  Matrix Multiply3/1 -> angleBtw2DVecs1/1(vec1)
  Constant6/1 -> Matrix Multiply3/2
  Matrix Multiply2/1 -> angleBtw2DVecs1/2(vec2)
  tan2Gr/1 -> Matrix Multiply1/1, Matrix Multiply3/1
  Subtract1/1 -> Terminator/1  "tanPitch"
  bdy2Inert/1 -> Matrix Multiply/1, Matrix Multiply2/1
  Gain/1 -> tanRoll/1  "tanRoll"
  Matrix Multiply/1 -> angleBtw2DVecs/2
  Constant4/1 -> Matrix Multiply1/2
  Matrix Multiply1/1 -> angleBtw2DVecs/1
  Constant2/1 -> Subtract/1
  angleBtw2DVecs/1 -> Subtract/2
  Constant3/1 -> Matrix Multiply/2
  Subtract/1 -> Gain/1

== system pathFollowingControllerExpStateMachineOpenWater_cl/pathFollowingControllerExpStateMachineOpenWater/desiredMoment/Wrap Correction ==
  note: output = mod(input-pi,2*pi)-pi
      | wraps output to -pi to pi
      |
      | ex) 1.5*pi will become -.5pi
      | 	and -1.5pi will become .5pi
      |
      | to visualize, plot the fuction above
  u : Inport
  Add1 : Sum  Inputs=+-
  Add2 : Sum  Inputs=+-
  Constant1 : Constant  Value=pi
  Constant2 : Constant  Value=2*pi
  Constant3 : Constant  Value=pi
  Mod : Math  Operator=mod  SignedPower=on  SaturateOnIntegerOverflow=on
  y : Outport  VectorParamsAs1DForOutWhenUnconnected=off
  wires:
  Add2/1 -> y/1
  Constant3/1 -> Add2/2
  Mod/1 -> Add2/1  "always_pos"
  Constant2/1 -> Mod/2
  Add1/1 -> Mod/1
  Constant1/1 -> Add1/2
  u/1 -> Add1/1

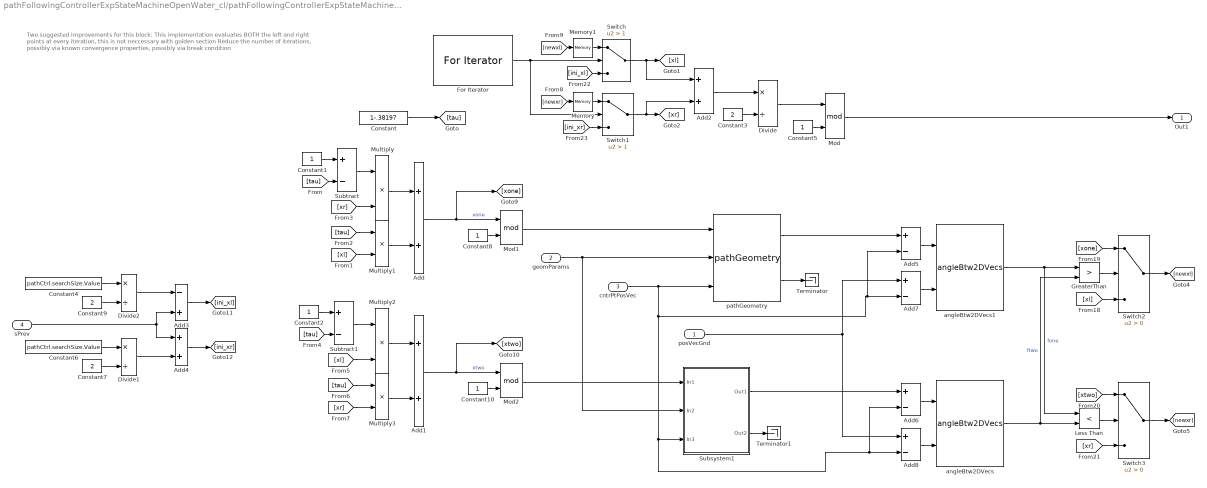
== system pathFollowingControllerExpStateMachineOpenWater_cl/pathFollowingControllerExpStateMachineOpenWater/courseFollowExp/GoldenSectionPathSearch/GoldenSectionSimulink ==
  note: Two suggested improvements for this block:
      | This implementation evaluates BOTH the left and right points at every iteration, this is not neccessary with golden section
      | Reduce the number of iterations, possibly via known convergence properties, possibly via break condition
  posVecGnd : Inport
  geomParams : Inport  Port=2
  cntrPtPosVec : Inport  Port=3
  sPrev : Inport  Port=4
  Add{,1..2,4} (4 alike) : Sum
  Add3 : Sum  Inputs=-+
  Add{5..8} (4 alike) : Sum  Inputs=+-
  Constant : Constant  Value=1-.38197
  Constant{1..2,5,8,10} (5 alike) : Constant
  Constant3 : Constant  Value=2
  Constant4 : Constant  Value=pathCtrl.searchSize.Value
  Constant6 : Constant  Value=pathCtrl.searchSize.Value
  Constant7 : Constant  Value=2
  Constant9 : Constant  Value=2
  Divide : Product  Inputs=*/
  Divide1 : Product  Inputs=*/
  Divide2 : Product  Inputs=*/
  For Iterator : ForIterator  IterationLimit=25
  GreaterThan : RelationalOperator  Operator=>  OutDataTypeStr=boolean  RndMeth=Simplest
  Less Than : RelationalOperator  Operator=<  OutDataTypeStr=boolean  RndMeth=Simplest
  Memory : Memory  InheritSampleTime=on
  Memory1 : Memory  InheritSampleTime=on
  Mod : Math  Operator=mod  SignedPower=on  SaturateOnIntegerOverflow=on
  Mod1 : Math  Operator=mod  SignedPower=on  SaturateOnIntegerOverflow=on
  Mod2 : Math  Operator=mod  SignedPower=on  SaturateOnIntegerOverflow=on
  Multiply{,1..3} (4 alike) : Product
  Subsystem1 : Subsystem
  Subtract : Sum  Inputs=+-
  Subtract1 : Sum  Inputs=+-
  Switch : Switch  Criteria=u2 > Threshold  Threshold=1
  Switch1 : Switch  Criteria=u2 > Threshold  Threshold=1
  Switch2 : Switch  Criteria=u2 > Threshold
  Switch3 : Switch  Criteria=u2 > Threshold
  Terminator : Terminator
  Terminator1 : Terminator
  angleBtw2DVecs : angleBtw2Vecs_ul/angleBtw2DVecs  SystemSampleTime=-1  Latency=0  AutoFrameSizeCalculation=off
  angleBtw2DVecs1 : angleBtw2Vecs_ul/angleBtw2DVecs  SystemSampleTime=-1  Latency=0  AutoFrameSizeCalculation=off
  pathGeometry : pathGeometry_ul/pathGeometry  SystemSampleTime=-1  Latency=0  AutoFrameSizeCalculation=off
  Out1 : Outport
  wires:
  Add8/1 -> angleBtw2DVecs/2
  Multiply1/1 -> Add/2
  Switch3/1 -> [newxr]
  [ini_xl] -> Switch/3
  Mod/1 -> Out1/1
  Divide2/1 -> Add3/1
  Switch2/1 -> [newxl]
  pathGeometry/2 -> Terminator/1
  [newxl] -> Memory1/1
  Constant6/1 -> Divide1/1
  Add6/1 -> angleBtw2DVecs/1
  Constant10/1 -> Mod2/2
  Add2/1 -> Divide/1
  [xl] -> Switch2/3
  [xr] -> Switch3/3
  Divide/1 -> Mod/1
  [xl] -> Multiply2/2
  Multiply3/1 -> Add1/2
  Add5/1 -> angleBtw2DVecs1/1
  sPrev/1 -> Add3/2, Add4/1
  Less Than/1 -> Switch3/2
  Constant3/1 -> Divide/2
  Add4/1 -> [ini_xr]
  Constant9/1 -> Divide2/2
  [xr] -> Multiply/2
  Add3/1 -> [ini_xl]
  Divide1/1 -> Add4/2
  Mod1/1 -> pathGeometry/1
  Memory/1 -> Switch1/1
  [newxr] -> Memory/1
  Add7/1 -> angleBtw2DVecs1/2
  [tau] -> Multiply1/1
  [xone] -> Switch2/1
  [ini_xr] -> Switch1/3
  angleBtw2DVecs1/1 -> GreaterThan/1, Less Than/1  "fone"
  Constant4/1 -> Divide2/1
  Mod2/1 -> Subsystem1/1(In1)
  Multiply2/1 -> Add1/1
  Switch1/1 -> [xr], Add2/2
  Constant/1 -> [tau]
  Add/1 -> Mod1/1, [xone]  "xone"
  For Iterator/1 -> Switch/2, Switch1/2
  Memory1/1 -> Switch/1
  [tau] -> Multiply3/1
  [tau] -> Subtract/2
  [xtwo] -> Switch3/1
  Multiply/1 -> Add/1
  [xl] -> Multiply1/2
  Subsystem1/2(Out2) -> Terminator1/1
  Subtract/1 -> Multiply/1
  Constant7/1 -> Divide1/2
  Add1/1 -> Mod2/1, [xtwo]  "xtwo"
  [tau] -> Subtract1/2
  angleBtw2DVecs/1 -> Less Than/2, GreaterThan/2  "ftwo"
  Constant5/1 -> Mod/2
  Constant1/1 -> Subtract/1
  posVecGnd/1 -> Add7/1, Add8/1
  GreaterThan/1 -> Switch2/2
  pathGeometry/1 -> Add5/1
  Constant8/1 -> Mod1/2
  [xr] -> Multiply3/2
  Subsystem1/1(Out1) -> Add6/1
  Constant2/1 -> Subtract1/1
  geomParams/1 -> Subsystem1/2(In2), pathGeometry/2
  Switch/1 -> [xl], Add2/1
  cntrPtPosVec/1 -> pathGeometry/3, Add7/2, Add5/2, Subsystem1/3(In3), Add8/2, Add6/2
  Subtract1/1 -> Multiply2/1

== system pathFollowingControllerExpStateMachineOpenWater_cl/pathFollowingControllerExpStateMachineOpenWater/desiredMoment/TangentRollCalculation/angleBtw2DVecs1 ==
  vec1 : Inport
  vec2 : Inport  Port=2
  Abs : Abs
  Atan2 : Trigonometry  Operator=atan2
  Cross Product : vrlib/Utilities/Cross Product
      settings: SourceProductBaseCode=VR
  Dot Product : DotProduct  InputSameDT=on  OutDataTypeStr=Inherit: Inherit via internal rule
  Dot Product1 : DotProduct  InputSameDT=on  OutDataTypeStr=Inherit: Inherit via internal rule
  Sqrt : Sqrt  SaturateOnIntegerOverflow=on
  angle : Outport  VectorParamsAs1DForOutWhenUnconnected=off
  wires:
  Sqrt/1 -> Atan2/1
  Dot Product1/1 -> Sqrt/1
  Abs/1 -> angle/1
  Dot Product/1 -> Atan2/2
  Cross Product/1 -> Dot Product1/2, Dot Product1/1
  vec2/1 -> Dot Product/2, Cross Product/1
  vec1/1 -> Cross Product/2, Dot Product/1
  Atan2/1 -> Abs/1

== system pathFollowingControllerExpStateMachineOpenWater_cl/pathFollowingControllerExpStateMachineOpenWater/courseFollowExp/GoldenSectionPathSearch/GoldenSectionSimulink/Subsystem1 ==
  In1 : Inport
  In2 : Inport  Port=2
  In3 : Inport  Port=3
  pathGeometry : pathGeometry_ul/pathGeometry  SystemSampleTime=-1  Latency=0  AutoFrameSizeCalculation=off
  Out1 : Outport  VectorParamsAs1DForOutWhenUnconnected=off
  Out2 : Outport  Port=2  VectorParamsAs1DForOutWhenUnconnected=off
  wires:
  pathGeometry/2 -> Out2/1
  In1/1 -> pathGeometry/1
  In3/1 -> pathGeometry/3
  pathGeometry/1 -> Out1/1
  In2/1 -> pathGeometry/2

== matlab function pathFollowingControllerExpStateMachineOpenWater_cl/pathFollowingControllerExpStateMachineOpenWater/courseFollowExp/GoldenSectionPathSearch/GoldenSectionMATLAB ==
  data: posVec input; sNext output; sPrev input; pathCntrPosVecGnd input; pathVarTol parameter; searchWidth parameter; geomParams input
function sNext = fcn(posVec,sPrev,pathCntrPosVecGnd, pathVarTol, searchWidth, geomParams)
% I wrote this function on 4/22/2020 when attempting to figure out some
% issues with numerical stiffness.  Turns out that althought the profiler
% was telling me the problem was with the simulink in the equivalent
% subsystem, that was a lie.  Anyways, I thought I should leave this here
% anyways just in case anyone wants to reference it.  Note that this
% implementation doesn't allow for different paths without changing
% function J below.  Which isn't great for a long term solution, so don't
% just use this as-is if you want to go to a matlab-based golden section
% implementation in the future. Also, I think there are some hard-coded
% numbers in the mask in the model, so fix that.  Finally, note that even
% though the "equivalent" simulink implementation has some inefficiencies
% that this code doesnt (as noted in the simulink implementation), there
% doesn't appear to be a siginificant difference in run times, although I
% haven't done a thorough study. -Mitchell

% phi = (sqrt(5) + 1) / 2;
% gr = 1/((1/phi)+1);
% gr = 0.618033988749895;
x1 = sPrev - searchWidth/2;
x4 = sPrev + searchWidth/2;
x2 = x4 - (x4-x1)*0.618033988749895;
x3 = x1 + (x4-x1)*0.618033988749895;
% J1 = J(x1,posVec,geomParams,pathCntrPosVecGnd);
J2 = J(x2,posVec,geomParams,pathCntrPosVecGnd);
J3 = J(x3,posVec,geomParams,pathCntrPosVecGnd);
% J4 = J(x4,posVec,geomParams,pathCntrPosVecGnd);
% JL =JFunc(xL);
% JR = JFunc(xR);
% plot([x1 x2 x3 x4],[J1 J2 J3 J4])
for ii = 1:100 
    if J2<J3
        x4 = x3;
%         J4 = J(x4,posVec,geomParams,pathCntrPosVecGnd);
        x3 = x2;
        J3 = J2;
        x2 = x4 - (x4-x1)*0.618033988749895;
        J2 = J(x2,posVec,geomParams,pathCntrPosVecGnd);
    else
        x1 = x2;
%         J1 = J(x1,posVec,geomParams,pathCntrPosVecGnd);
        x2 = x3;
        J2 = J3;
        x3 = x1 + (x4-x1)*0.618033988749895;
        J3 = J(x3,posVec,geomParams,pathCntrPosVecGnd);
    end
    if x4-x1<pathVarTol/2
        break
    end
end
sNext = mod((x4+x1)/2,1);
end

function val = J(sTest,posVec,geomParams,pathCntr)
az = atan2(posVec(2),posVec(1));
el = atan2(posVec(3),sqrt(posVec(1)^2+posVec(2)^2));
pathPosVec = lemOfBooth(sTest,geomParams,pathCntr);
azP = atan2(pathPosVec(2),pathPosVec(1));
elP = atan2(pathPosVec(3),sqrt(pathPosVec(1)^2+pathPosVec(2)^2));
val = (az-azP)^2+(el-elP)^2;
end

== matlab function pathFollowingControllerExpStateMachineOpenWater_cl/pathFollowingControllerExpStateMachineOpenWater/pathShapeScaler/MATLAB Function1 ==
  data: r input; basisParams output
function basisParams = fcn(r)

h = 2*asin(2/2/r );  w = 2*asin(6/2/r );                              %   rad - Path width/height
[a,b] = boothParamConversion(w,h);

basisParams = [a,b,deg2rad(35),0*pi/180,r-.1];

== matlab function pathFollowingControllerExpStateMachineOpenWater_cl/pathFollowingControllerExpStateMachineOpenWater/MATLAB Function ==
  data: t input; wnchGain output; vSat input
function wnchGain   = fcn(t,vSat)
wnchGain = 0;
if t< 24 || t>150
    wnchGain = 0;
else
    wnchGain = .0005*(t-24)^2;
end

% if wnchGain >= vSat
%     wnchGain = vSat;
% end
